simulink model "Lab_Encoder"  (R2026a)
settings: Solver=FixedStepDiscrete  StopTime=inf  FixedStep=0.001
undefined symbols (not defined in the file or in its folder): Blocking, Non
libraries: amg_usbconverter_n_connect_lib x2
settings Model: Creator=pboon  LastModifiedBy=Lenovo LOQ

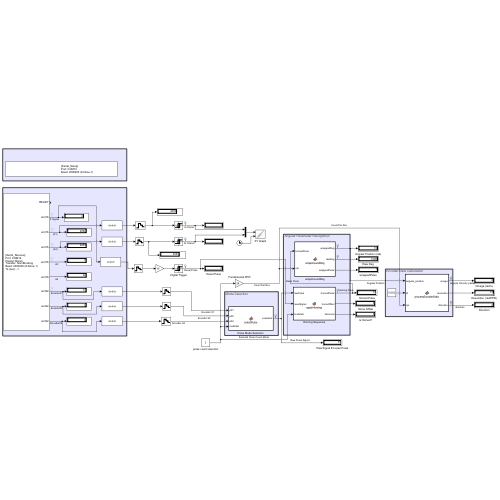
[thumbnail: Simulink's stored preview of the top-level diagram]
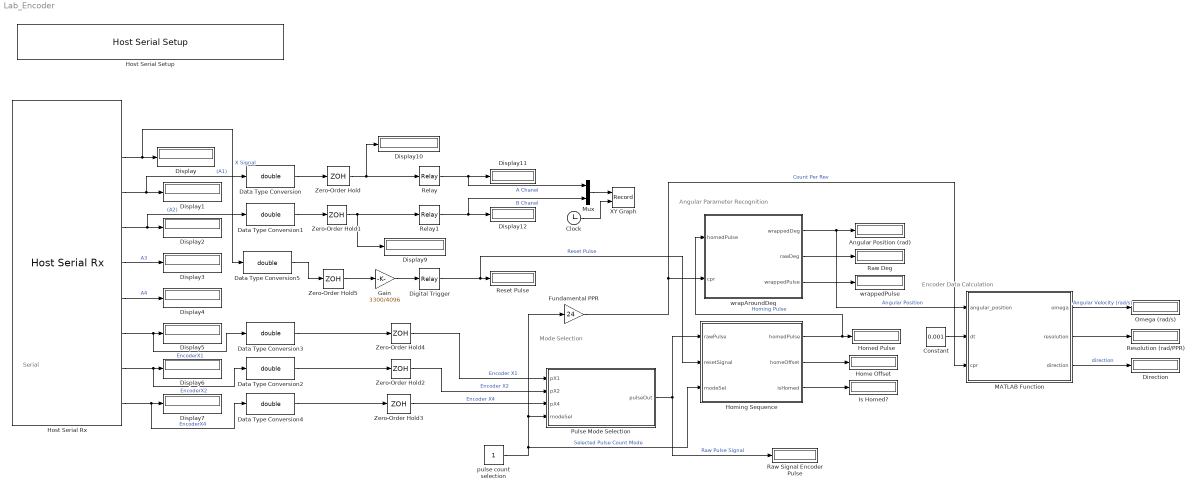
== system Lab_Encoder ==
  note: Mode Selection
  note: Encoder Data Calculation
  note: Angular Parameter Recognition
  note: Serial
  Angular Position (rad) : Display
  Clock : Clock
  Constant : Constant  Value=0.001
  Data Type Conversion{,1..5} (6 alike) : DataTypeConversion  OutDataTypeStr=double  SaturateOnIntegerOverflow=off  RndMeth=Floor
  Digital Trigger : Relay  OnSwitchValue=3200  OffSwitchValue=30
  Direction : Display
  Display{,1..7,9..12} (12 alike) : Display
  Fundamental PPR : Gain  Gain=24
  Gain : Gain  Gain=3300/4096
  Home Offset : Display
  Homed Pulse : Display
  Homing Sequence : MATLAB Function  TreatAsAtomicUnit=on
  Host Serial Rx : amg_usbconverter_n_connect_lib/Host Serial Rx  conf=rx  port=COM12  baudrate=2000000  databits=8  parity=None  stopbit=1  flowcontrol=None  transfer=Non-Blocking  timeout=5  packetmode=Binary  enableinitialvalues=off  initialvalues=[]  binheader='25'  binterminator='4E 4E'  porttype_double=0  porttype_single=0  porttype_int8=0  porttype_uint8=0  porttype_int16=0  porttype_uint16=5  porttype_int32=0  porttype_uint32=3  asciiformat='%d,%f'  rx_asciiterminator="CRLF (0x0D 0x0A - \"\\r\\n\")"  tx_asciiterminator="CRLF (0x0D 0x0A - \"\\r\\n\")"  sampletime=0.001  enablecustomportlabel=off  cinputportlabel=0  coutputportlabel=A  portpinstr=0  blockid=HostSerialRx  inputporttype=[]  inputportwidth=[]  inputportlabel={}  outputporttype=[3 5 5 5 5 5 7 7 7]  outputportwidth=[1 1 1 1 1 1 1 1 1]  outputportlabel={'READY','uint16','uint16','uint16','uint16','uint16','uint32','uint32','uint32'}  compat=0  optionstring=[]  autoport='COM12'
  Host Serial Setup : amg_usbconverter_n_connect_lib/Host Serial Setup  conf=setup  port=COM12  baudrate=2000000  databits=8  parity=None  stopbit=1  flowcontrol=None  transfer=Blocking  timeout=2  packetmode=Binary  initialvalues=[]  binheader='7E 7E'  binterminator='03 03'  porttype_double=0  porttype_single=1  porttype_int8=0  porttype_uint8=0  porttype_int16=0  porttype_uint16=0  porttype_int32=0  porttype_uint32=2  asciiformat='%d %u %x'  rx_asciiterminator="CRLF (0x0D 0x0A - \"\\r\\n\")"  tx_asciiterminator="CRLF (0x0D 0x0A - \"\\r\\n\")"  sampletime=-1  enablecustomportlabel=off  cinputportlabel=0  coutputportlabel=A  portpinstr=0  blockid=HostSerialSetup  inputporttype=[]  inputportwidth=[]  inputportlabel={}  outputporttype=[]  outputportwidth=[]  outputportlabel={}  compat=0  optionstring=[]  autoport='COM12'
  Is Homed? : Display
  MATLAB Function : MATLAB Function  TreatAsAtomicUnit=on
  Mux : Mux  Inputs=2
  Omega (rad/s) : Display
  "Pulse Mode Selection " : MATLAB Function  TreatAsAtomicUnit=on
  Raw Deg : Display
  Raw Signal Encoder Pulse : Display
  Relay : Relay  OnSwitchValue=3200  OffSwitchValue=30
  Relay1 : Relay  OnSwitchValue=3200  OffSwitchValue=30
  Reset Pulse : Display
  Resolution (rad/PPR) : Display
  XY Graph : Record  NumPorts=2.0  FileSettingsInternal="{\"entries\":[{\"content\":{\"excelSettings\":{\"content\":{},\"type\":\"Streamout.ExcelSettings\"},\"parquetSettings\":{\"content\":{},\"type\":\"Streamout.ParquetSettings\"}},\"type\":\"Streamout.FileSettingStorage\",\"uuid\":\"\"}],\"packageUris\":[\"http:\\/\\/schema.mathworks.com\\/mf0\\/streamout_blocks\\/R2020a\"],\"version\":\"1.0\"}"  FrameSettings=[0, 0]  Layout=[1 1]  SignalsInternal="{\"entries\":[{\"content\":{\"signals\":[{\"content\":{\"blockPath\":[],\"dimensions\":[2],\"domain\":\"\",\"hasChildren\":true,\"lineColor\":\"#edb120\",\"lineWidth\":2,\"port\":1,\"sid\":[\"\"],\"signalID\":1,\"signalName\":\"Mux\"},\"type\":\"RecordBlkView.Signal\",\"uuid\":\"\"},{\"content\":{\"blockPath\":[],\"channel\":[1],\"dimensions\":[2],\"domain\":\"\",\"lineColor\":\"#0072bd\",\"lineWidth\":2,\"parentID\":1,\"plots\":[ 1 ],\"port\":1,\"sid\":[\"\"],\"signalID\":2,\"signalName\":\"Mux\"},\"type\":\"RecordBlkView.Signal\",\"uuid\":\"\"},{\"content\":{\"blockPath\":[],\"dimensions\":[1],\"domain\":\"\",\"lineColor\":\"#139fff\",\"port\":2,\"sid\":[\"\"],\"signalID\":3,\"signalName\":\"Clock\"},\"type\":\"RecordBlkView.Signal\",\"uuid\":\"\"},{\"content\":{\"blockPath\":[],\"channel\":[2],\"dimensions\":[2],\"domain\":\"\",\"lineColor\":\"#edb120\",\"lineWidth\":2,\"parentID\":1,\"plots\":[ 1 ],\"port\":1,\"sid\":[\"\"],\"signalID\":4,\"signalName\":\"Mux\"},\"type\":\"RecordBlkView.Signal\",\"uuid\":\"\"}]},\"type\":\"RecordBlkView.InputSignals\",\"uuid\":\"\"}],\"packageUris\":[\"http:\\/\\/schema.mathworks.com\\/mf0\\/streamout_blocks\\/R2020a\"],\"version\":\"1.0\"}"  CompatibilityTag=XY
  Zero-Order Hold{,1..5} (6 alike) : ZeroOrderHold  SampleTime=0.001
  pulse count selection : Constant
  wrapAroundDeg : MATLAB Function  TreatAsAtomicUnit=on
  wrappedPulse : Display
  wires:
  Host Serial Rx/2 -> Data Type Conversion5/1, Display/1  "X Signal"
  Host Serial Rx/3 -> Data Type Conversion/1, Display1/1  "(A1)"
  Host Serial Rx/4 -> Data Type Conversion1/1, Display2/1  "(A2)"
  Host Serial Rx/5 -> Display3/1  "A3"
  Host Serial Rx/6 -> Display4/1  "A4"
  Host Serial Rx/7 -> Data Type Conversion3/1, Display5/1  "EncoderX1"
  Host Serial Rx/8 -> Data Type Conversion2/1, Display6/1  "EncoderX2"
  Host Serial Rx/9 -> Data Type Conversion4/1, Display7/1  "EncoderX4"
  Data Type Conversion/1 -> Zero-Order Hold/1
  Data Type Conversion1/1 -> Zero-Order Hold1/1
  Zero-Order Hold/1 -> Relay/1, Display10/1
  Zero-Order Hold1/1 -> Relay1/1, Display9/1
  Relay/1 -> Mux/1, Display11/1  "A Chanel"
  Relay1/1 -> Mux/2, Display12/1  "B Chanel"
  Data Type Conversion2/1 -> Zero-Order Hold2/1
  Data Type Conversion4/1 -> Zero-Order Hold3/1
  Data Type Conversion3/1 -> Zero-Order Hold4/1
  Data Type Conversion5/1 -> Zero-Order Hold5/1
  Zero-Order Hold5/1 -> Gain/1
  Gain/1 -> Digital Trigger/1
  Digital Trigger/1 -> Homing Sequence/2(resetSignal), Reset Pulse/1  "Reset Pulse"
  Homing Sequence/1(homedPulse) -> wrapAroundDeg/1(homedPulse), Homed Pulse/1  "Homing Pulse"
  Homing Sequence/2(homeOffset) -> Home Offset/1
  Homing Sequence/3(isHomed) -> Is Homed?/1
  Zero-Order Hold2/1 -> "Pulse Mode Selection "/2(pX2)  "Encoder X2"
  Zero-Order Hold3/1 -> "Pulse Mode Selection "/3(pX4)  "Encoder X4"
  "Pulse Mode Selection "/1(pulseOut) -> Homing Sequence/1(rawPulse), Raw Signal Encoder Pulse/1  "Raw Pulse Signal"
  Zero-Order Hold4/1 -> "Pulse Mode Selection "/1(pX1)  "Encoder X1"
  pulse count selection/1 -> Fundamental PPR/1, "Pulse Mode Selection "/4(modeSel), Homing Sequence/3(modeSel)  "Selected Pulse Count Mode"
  wrapAroundDeg/1(wrappedDeg) -> Angular Position (rad)/1, MATLAB Function/1(angular_position)  "Angular Position"
  wrapAroundDeg/2(rawDeg) -> Raw Deg/1
  wrapAroundDeg/3(wrappedPulse) -> wrappedPulse/1
  Fundamental PPR/1 -> wrapAroundDeg/2(cpr), MATLAB Function/3(cpr)  "Count Per Rev"
  Constant/1 -> MATLAB Function/2(dt)
  MATLAB Function/2(resolution) -> Resolution (rad/PPR)/1
  MATLAB Function/3(direction) -> Direction/1  "direction"
  Mux/1 -> XY Graph/1
  Clock/1 -> XY Graph/2
  MATLAB Function/1(omega) -> Omega (rad/s)/1  "Angular Velocity (rad/s)"

== matlab function Lab_Encoder/Homing Sequence ==
  data: rawPulse input; resetSignal input; modeSel input; homedPulse output; homeOffset output; isHomed output
function [homedPulse, homeOffset, isHomed] = applyHoming(rawPulse, resetSignal, modeSel)
    persistent savedOffset prevReset homedFlag prevMode

    if isempty(savedOffset)
        savedOffset = 0;
        prevReset = 0;
        homedFlag = false;
        prevMode = modeSel;
    end

    % ตรวจจับการเปลี่ยนโหมดการนับ Pulse เพื่อล้าง Home Offset
    if modeSel ~= prevMode
        savedOffset = 0;
        homedFlag = false;
        prevMode = modeSel;
    end

    % ตรวจจับ Rising Edge เมื่อกดปุ่ม Reset
    if (resetSignal > 0) && (prevReset == 0)
        savedOffset = rawPulse;
        homedFlag = true;
    end

    prevReset = resetSignal;

    homeOffset = savedOffset;
    isHomed = homedFlag;
    homedPulse = rawPulse - savedOffset;
end

== matlab function Lab_Encoder/Pulse Mode Selection  ==
  data: pX1 input; pulseOut output; pX2 input; pX4 input; modeSel input
function pulseOut = selectPulse(pX1, pX2, pX4, modeSel)
    switch modeSel
        case 1
            pulseOut = pX1;
        case 2
            pulseOut = pX2;
        case 4
            pulseOut = pX4;
        otherwise
            pulseOut = pX1;
    end
end

== matlab function Lab_Encoder/wrapAroundDeg ==
  data: homedPulse input; wrappedDeg output; cpr input; rawDeg output; wrappedPulse output
function [wrappedDeg, rawDeg, wrappedPulse] = wrapAroundDeg(homedPulse, cpr)
    if cpr > 0
        % คำนวณมุมสะสมจริงแบบต่อเนื่อง (สะสมเกิน 360 องศาได้)
        rawDeg = (double(homedPulse) / double(cpr)) * 360.0;
        
        % จำกัดขอบเขตพัลส์ให้อยู่ในช่วง 0 ถึง (cpr - 1)
        wrappedPulse = mod(double(homedPulse), double(cpr));
        
        % จำกัดขอบเขตมุมให้อยู่ในช่วง 0 ถึง 360 องศา
        wrappedDeg = mod(rawDeg, 360.0);
    else
        rawDeg = 0.0;
        wrappedPulse = 0;
        wrappedDeg = 0.0;
    end
end

== matlab function Lab_Encoder/MATLAB Function ==
  data: angular_position input; dt input; omega output; cpr input; resolution output; direction output
function [omega, resolution, direction] = processEncoderData(angular_position, dt, cpr)
    persistent prev_position last_omega last_direction pulse_timer
    if isempty(prev_position)
        prev_position = angular_position;
        last_omega = 0;
        last_direction = 0;
        pulse_timer = 0;
    end

    d_theta = angular_position - prev_position;
    pulse_timer = pulse_timer + dt;

    if d_theta ~= 0
        % คำนวณความเร็วทันทีเมื่อตำแหน่งเปลี่ยน โดยใช้เวลาที่สะสมจริง
        instant_omega = d_theta / pulse_timer;
        
        % กรองค่าความเร็วที่สูงเกินขีดจำกัดทางกายภาพ (Spike ป้องกันค่ากระโดด)
        if abs(instant_omega) < 1000 
            last_omega = instant_omega;
        end
        
        prev_position = angular_position;
        pulse_timer = 0;
        
        if d_theta > 0
            last_direction = 1;
        else
            last_direction = -1;
        end
    else
        % ถ้าเวลาผ่านไปนานเกิน 0.1 วินาทีแล้วตำแหน่งยังไม่เปลี่ยน ให้ปรับความเร็วเป็น 0
        if pulse_timer > 0.1
            last_omega = 0;
            last_direction = 0;
        end
    end

    omega = last_omega;
    direction = last_direction;

    resolution_deg = 360 / cpr;
    resolution_rad = 2 * pi / cpr;
    resolution = [resolution_deg, resolution_rad];
end
